simulink model "non_linear_model"  (R2023b)
settings: Solver=VariableStepAuto  StartTime=0.0  StopTime=6  RelTol=1e-3
values from neighbouring files (symbols this model uses):
  den_mag_C = Gden{1}    [Controllo_un_anello_v2.m]
  num_mag_C = Gnum{1}    [Controllo_un_anello_v2.m]
  Upper_bound_V = 23    [Controllo_un_anello_v2.m]
  x1_eq = 0.0044    [Controllo_un_anello_v2.m]
undefined symbols (not defined in the file or in its folder): k_mag, ki, kp, Lc, m, Rtot, theta, ueq, y0
libraries: slpidlib x2, SignalEditorBlockLib x1
settings Model: Creator=lollo  LastModifiedBy=lollo

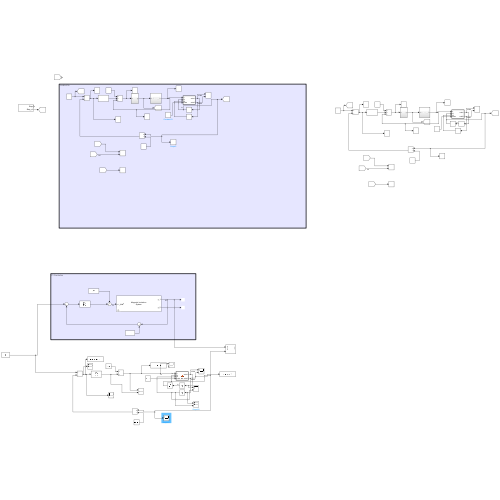
[thumbnail: Simulink's stored preview of the top-level diagram]
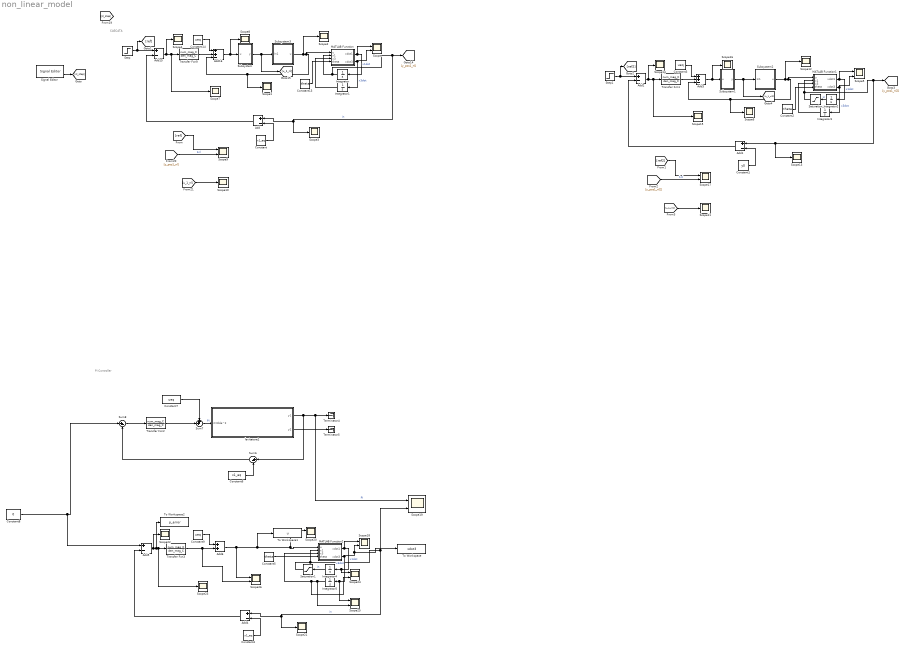
== system non_linear_model ==
  note: CASCATA
  note: PI Controller
  Add{,1..2,4..5,15} (6 alike) : Sum  Inputs=+-
  Add16 : Sum  Inputs=++-
  Add3 : Sum  Inputs=++-
  Add6 : Sum
  Constant : Constant  Value=x1_eq
  Constant1 : Constant  Value=y0
  Constant13 : Constant  Value=theta
  Constant{3,7,9,14} (4 alike) : Constant  Value=ueq
  Constant2 : Constant  Value=theta
  Constant4 : Constant  Value=x1_eq
  Constant5 : Constant  Value=theta
  Constant6 : Constant  Value=x1_eq
  Constant8 : Constant  Value=0
  Integrator{,1..5} (6 alike) : Integrator
  MATLAB Function : MATLAB Function  TreatAsAtomicUnit=on
  MATLAB Function1 : MATLAB Function  TreatAsAtomicUnit=on
  MATLAB Function2 : MATLAB Function  TreatAsAtomicUnit=on
  Saturation : Saturate  UpperLimit=0.012  LowerLimit=0
  Saturation1 : Saturate  UpperLimit=0.012  LowerLimit=0
  Scope{,5,9,17..20,24..26} (10 alike) : Scope  NumInputPorts=2
  Scope{1..4,6..8,10..16,21..23} (17 alike) : Scope
  Signal Editor : SignalEditorBlockLib/Signal Editor  FileName=input_signal.mat  ActiveScenario=Scenario  ActiveSignal=Step_nl  IsBus=off  OutputBusObjectStr=Bus: BusObject  SampleTime=0  Interpolate=off  ZeroCross=off  OutputAfterFinalValue=Setting to zero  Unit=inherit  PreserveSignalName=on  ApplySigPropsToAllScenarios=on  ApplySigPropsToAllSignals=off
  Step : Step  After=0.001  SampleTime=0
  Step1 : Step  After=0.001  SampleTime=0
  Subsystem : Subsystem
  Subsystem1 : Subsystem
  Subsystem2 : Subsystem
  Subsystem3 : Subsystem
  Sum6 : Sum  Inputs=|+-
  Sum7 : Sum  Inputs=++|
  Sum8 : Sum  Inputs=|+-
  Terminator4 : Terminator
  Terminator5 : Terminator
  To Workspace : ToWorkspace  VariableName=xdot3  SaveFormat=Timeseries  SampleTime=-1
  To Workspace1 : ToWorkspace  VariableName=u  SaveFormat=Timeseries  SampleTime=-1
  To Workspace2 : ToWorkspace  VariableName=p_error  SaveFormat=Timeseries  SampleTime=-1
  Transfer Fcn{1..3,9} (4 alike) : TransferFcn  Numerator=num_mag_C  Denominator=den_mag_C
  levitatore2 : Subsystem  Description=|  mask{y1_0=0, y2_0=0}
      | Magnetic Levitation System.
      | The input is the squared current. The outputs are the position (y1) and the velocity (y2).
      mask prompts: y1_0 "Initial value for y1"; y2_0 "Initial value for y2"
      mask DialogControl DescTextVar Prompt: Magnetic Levitation System. The input is the squared current. The outputs are the position (y1) and the velocity (y2).
      mask Display:
      | disp('Magnetic Levitation\nSystem');
      | port_label('input', 1, 'i= i\_tilde^2', 'texmode', 'on');
      | port_label('output', 1, 'y_1');
      | port_label('output', 2, 'y_2');
  wires:
  [y_pos1_nl] -> Scope9/2  "1nl"
  Transfer Fcn9/1 -> Add16/2
  Integrator/1 -> Add/1, Scope3/1, [y_pos1_nl], MATLAB Function/2(x1)  "in"
  Add16/1 -> Scope8/1, Subsystem/1(u)
  Integrator1/1 -> MATLAB Function/3(x3)
  Constant14/1 -> Add16/1
  Constant13/1 -> MATLAB Function/4(theta)
  Subsystem/1(y) -> [u_1_nl], Subsystem3/1(In1)
  MATLAB Function/1(xdot1) -> Scope/1, Integrator/1  "x1dot"
  Add15/1 -> Scope4/1, Scope7/1, Transfer Fcn9/1
  MATLAB Function/2(xdot3) -> Scope/2, Integrator1/1  "x3dot"
  [u_1_nl] -> Scope10/1
  Subsystem3/1(u) -> Scope2/1, MATLAB Function/1(u), Scope1/1, Add16/3
  Signal Editor/2 -> [nl_step]
  [ref] -> Scope9/1
  Step/1 -> [ref], Add15/1
  Constant/1 -> Add/2
  Add/1 -> Add15/2
  Add1/1 -> Add2/2
  Constant1/1 -> Add1/2
  [ref2] -> Scope17/1
  Subsystem2/1(u) -> Scope12/1, MATLAB Function1/1(u), Scope6/1, Add3/3
  [u_1_nl2] -> Scope11/1
  MATLAB Function1/1(xdot1) -> Scope5/1, Integrator2/1  "x1dot"
  Add2/1 -> Scope14/1, Scope15/1, Transfer Fcn1/1
  Constant3/1 -> Add3/1
  MATLAB Function1/2(xdot3) -> Scope5/2, Integrator3/1  "x3dot"
  Add3/1 -> Scope16/1, Subsystem1/1(u)
  Subsystem1/1(y) -> [u_1_nl2], Subsystem2/1(In1)
  Constant2/1 -> MATLAB Function1/4(theta)
  [y_pos1_nl2] -> Scope17/2  "1nl"
  Step1/1 -> [ref2], Add2/1
  Integrator3/1 -> MATLAB Function1/3(x3)
  Transfer Fcn1/1 -> Add3/2
  Integrator2/1 -> Saturation/1  "in"
  Saturation/1 -> Scope13/1, Add1/1, [y_pos1_nl2], MATLAB Function1/2(x1)
  levitatore2/1(y1) -> Sum6/1, Scope19/1, Terminator4/1  "PI"
  Sum6/1 -> Sum8/2
  levitatore2/2(y2) -> Terminator5/1
  Sum7/1 -> levitatore2/1(i=itilde^2)  "PI"
  Constant8/1 -> Add5/1, Sum8/1
  Sum8/1 -> Transfer Fcn2/1
  Constant6/1 -> Sum6/2
  Transfer Fcn2/1 -> Sum7/2
  Constant7/1 -> Sum7/1
  Add4/1 -> Add5/2
  Constant4/1 -> Add4/2
  Add6/1 -> Scope26/1, To Workspace1/1, MATLAB Function2/1(u), Scope20/1
  MATLAB Function2/1(xdot1) -> Scope18/1, Scope24/1, Integrator4/1  "x1dot"
  Add5/1 -> Scope22/1, To Workspace2/1, Scope23/1, Transfer Fcn3/1
  Constant9/1 -> Add6/1
  MATLAB Function2/2(xdot3) -> To Workspace/1, Scope18/2, Scope25/1, Integrator5/1  "x3dot"
  Constant5/1 -> MATLAB Function2/4(theta)
  Saturation1/1 -> Add4/1, Scope21/1, Scope19/2, MATLAB Function2/2(x1)  "in"
  Integrator5/1 -> Scope25/2, Scope24/2, MATLAB Function2/3(x3)
  Transfer Fcn3/1 -> Scope26/2, Add6/2
  Integrator4/1 -> Saturation1/1  "in"

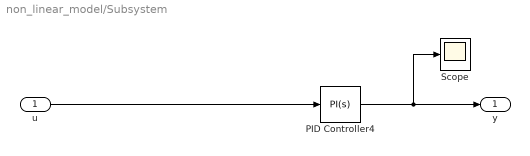
== system non_linear_model/Subsystem ==
  u : Inport
  PID Controller4 : slpidlib/PID Controller  Controller=PI  Form=Parallel  TimeDomain=Continuous-time  UseExternalTs=off  SampleTime=-1  IntegratorMethod=Forward Euler  FilterMethod=Forward Euler  ControllerParametersSource=internal  P=kp  I=ki  UseKiTs=off  D=0  N=100  UseFilter=on  TunerSelectOption=Transfer Function Based (PID Tuner App)  InitialConditionSource=internal  InitialConditionForIntegrator=0  InitialConditionForFilter=0  DifferentiatorICPrevScaledInput=0  ExternalReset=none  TrackingMode=off  Kt=1  LimitOutput=on  SatLimitsSource=internal  UpperSaturationLimit=Upper_bound_V  LowerSaturationLimit=0  LinearizeAsGain=on  AntiWindupMode=clamping  Kb=1  LimitIntegrator=off  UpperIntegratorSaturationLimit=inf  LowerIntegratorSaturationLimit=-inf  POutMin=[]  POutMax=[]  IOutMin=[]  IOutMax=[]  DOutMin=[]  DOutMax=[]  NOutMin=[]  NOutMax=[]  SumOutMin=[]  SumOutMax=[]  SaturationOutMin=[]  SaturationOutMax=[]  PParamMin=[]  PParamMax=[]  IParamMin=[]  IParamMax=[]  DParamMin=[]  DParamMax=[]  NParamMin=[]  NParamMax=[]  KbParamMin=[]  KbParamMax=[]  KtParamMin=[]  KtParamMax=[]  KbOutMin=[]  KbOutMax=[]  KtOutMin=[]  KtOutMax=[]  IntegratorOutMin=[]  IntegratorOutMax=[]  FilterOutMin=[]  FilterOutMax=[]  SumI1OutMin=[]  SumI1OutMax=[]  SumI2OutMin=[]  SumI2OutMax=[]  SumI3OutMin=[]  SumI3OutMax=[]  SumI4OutMin=[]  SumI4OutMax=[]  SumDOutMin=[]  SumDOutMax=[]  DifferentiatorOutMin=[]  DifferentiatorOutMax=[]  FilterDiffOutCoefMin=[]  FilterDiffOutCoefMax=[]  ReciprocalOutMin=[]  ReciprocalOutMax=[]  SumDenOutMin=[]  SumDenOutMax=[]  SumNumOutMin=[]  SumNumOutMax=[]  DivideOutMin=[]  DivideOutMax=[]  UdiffTsProdOutMin=[]  UdiffTsProdOutMax=[]  NTsProdOutMin=[]  NTsProdOutMax=[]  UintegralTsProdOutMin=[]  UintegralTsProdOutMax=[]  UngainTsProdOutMin=[]  UngainTsProdOutMax=[]  ClampingZeroOutDataTypeStr=Inherit: Inherit via back propagation  ClampingZeroOutMin=[]  ClampingZeroOutMax=[]  FilterDenConstantOutDataTypeStr=Inherit: Inherit via back propagation  FilterDenConstantOutMin=[]  FilterDenConstantOutMax=[]  PCopyOutDataTypeStr=Inherit: Inherit via back propagation  PCopyOutMin=[]  PCopyOutMax=[]  NCopyOutDataTypeStr=Inherit: Inherit via back propagation  NCopyOutMin=[]  NCopyOutMax=[]  IntegratorContinuousStateAttributes=''  IntegratorStateMustResolveToSignalObject=off  IntegratorRTWStateStorageClass=Auto  FilterContinuousStateAttributes=''  FilterStateMustResolveToSignalObject=off  FilterRTWStateStorageClass=Auto  ParallelPVariant=InternalParameters  IdealPVariant=Disabled  IVariant=InternalParameters  DVariant=Disabled  IntegratorVariant=Continuous  SatVariant=Enabled  AWVariant=ContClampingParallel  PCopyVariant=Disabled  TRVariant=Disabled  FdbkBlocksVariant=Forward  IdealPFdbkVariant=Disabled  SatFdbkVariant=Disabled  DerivativeFilterVariant=Disabled  NVariant=Disabled  NCopyVariant=Disabled_SignalSpec  FilterICVariant=Disabled  IntegratorICVariant=InternalICs  ExternalResetVariant=Disabled  TRSumVariant=Passthrough  SumFdbkVariant=Disabled  SumVariant=Sum_PI  TsampFilterVariant=InternalTs  TsampNgainVariant=Passthrough  TsampIntegralVariant=Disabled_SignalSpec  ExternalSaturationOutDataTypeStr=Inherit: Same as second input
  Scope : Scope
  y : Outport
  wires:
  PID Controller4/1 -> Scope/1, y/1
  u/1 -> PID Controller4/1

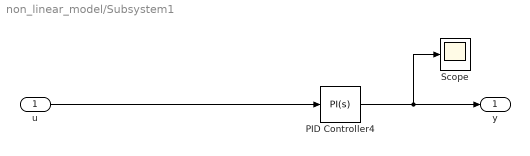
== system non_linear_model/Subsystem1 ==
  u : Inport
  PID Controller4 : slpidlib/PID Controller  Controller=PI  Form=Parallel  TimeDomain=Continuous-time  UseExternalTs=off  SampleTime=-1  IntegratorMethod=Forward Euler  FilterMethod=Forward Euler  ControllerParametersSource=internal  P=kp  I=ki  UseKiTs=off  D=0  N=100  UseFilter=on  TunerSelectOption=Transfer Function Based (PID Tuner App)  InitialConditionSource=internal  InitialConditionForIntegrator=0  InitialConditionForFilter=0  DifferentiatorICPrevScaledInput=0  ExternalReset=none  TrackingMode=off  Kt=1  LimitOutput=on  SatLimitsSource=internal  UpperSaturationLimit=Upper_bound_V  LowerSaturationLimit=0  LinearizeAsGain=on  AntiWindupMode=clamping  Kb=1  LimitIntegrator=off  UpperIntegratorSaturationLimit=inf  LowerIntegratorSaturationLimit=-inf  POutMin=[]  POutMax=[]  IOutMin=[]  IOutMax=[]  DOutMin=[]  DOutMax=[]  NOutMin=[]  NOutMax=[]  SumOutMin=[]  SumOutMax=[]  SaturationOutMin=[]  SaturationOutMax=[]  PParamMin=[]  PParamMax=[]  IParamMin=[]  IParamMax=[]  DParamMin=[]  DParamMax=[]  NParamMin=[]  NParamMax=[]  KbParamMin=[]  KbParamMax=[]  KtParamMin=[]  KtParamMax=[]  KbOutMin=[]  KbOutMax=[]  KtOutMin=[]  KtOutMax=[]  IntegratorOutMin=[]  IntegratorOutMax=[]  FilterOutMin=[]  FilterOutMax=[]  SumI1OutMin=[]  SumI1OutMax=[]  SumI2OutMin=[]  SumI2OutMax=[]  SumI3OutMin=[]  SumI3OutMax=[]  SumI4OutMin=[]  SumI4OutMax=[]  SumDOutMin=[]  SumDOutMax=[]  DifferentiatorOutMin=[]  DifferentiatorOutMax=[]  FilterDiffOutCoefMin=[]  FilterDiffOutCoefMax=[]  ReciprocalOutMin=[]  ReciprocalOutMax=[]  SumDenOutMin=[]  SumDenOutMax=[]  SumNumOutMin=[]  SumNumOutMax=[]  DivideOutMin=[]  DivideOutMax=[]  UdiffTsProdOutMin=[]  UdiffTsProdOutMax=[]  NTsProdOutMin=[]  NTsProdOutMax=[]  UintegralTsProdOutMin=[]  UintegralTsProdOutMax=[]  UngainTsProdOutMin=[]  UngainTsProdOutMax=[]  ClampingZeroOutDataTypeStr=Inherit: Inherit via back propagation  ClampingZeroOutMin=[]  ClampingZeroOutMax=[]  FilterDenConstantOutDataTypeStr=Inherit: Inherit via back propagation  FilterDenConstantOutMin=[]  FilterDenConstantOutMax=[]  PCopyOutDataTypeStr=Inherit: Inherit via back propagation  PCopyOutMin=[]  PCopyOutMax=[]  NCopyOutDataTypeStr=Inherit: Inherit via back propagation  NCopyOutMin=[]  NCopyOutMax=[]  IntegratorContinuousStateAttributes=''  IntegratorStateMustResolveToSignalObject=off  IntegratorRTWStateStorageClass=Auto  FilterContinuousStateAttributes=''  FilterStateMustResolveToSignalObject=off  FilterRTWStateStorageClass=Auto  ParallelPVariant=InternalParameters  IdealPVariant=Disabled  IVariant=InternalParameters  DVariant=Disabled  IntegratorVariant=Continuous  SatVariant=Enabled  AWVariant=ContClampingParallel  PCopyVariant=Disabled  TRVariant=Disabled  FdbkBlocksVariant=Forward  IdealPFdbkVariant=Disabled  SatFdbkVariant=Disabled  DerivativeFilterVariant=Disabled  NVariant=Disabled  NCopyVariant=Disabled_SignalSpec  FilterICVariant=Disabled  IntegratorICVariant=InternalICs  ExternalResetVariant=Disabled  TRSumVariant=Passthrough  SumFdbkVariant=Disabled  SumVariant=Sum_PI  TsampFilterVariant=InternalTs  TsampNgainVariant=Passthrough  TsampIntegralVariant=Disabled_SignalSpec  ExternalSaturationOutDataTypeStr=Inherit: Same as second input
  Scope : Scope
  y : Outport
  wires:
  PID Controller4/1 -> Scope/1, y/1
  u/1 -> PID Controller4/1

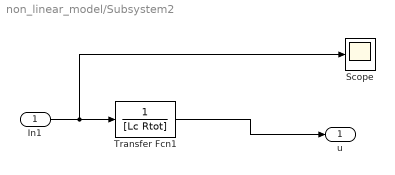
== system non_linear_model/Subsystem2 ==
  In1 : Inport
  Scope : Scope
  Transfer Fcn1 : TransferFcn  Denominator=[Lc Rtot]
  u : Outport
  wires:
  In1/1 -> Scope/1, Transfer Fcn1/1
  Transfer Fcn1/1 -> u/1

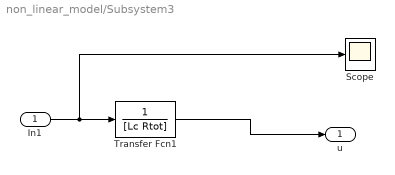
== system non_linear_model/Subsystem3 ==
  In1 : Inport
  Scope : Scope
  Transfer Fcn1 : TransferFcn  Denominator=[Lc Rtot]
  u : Outport
  wires:
  In1/1 -> Scope/1, Transfer Fcn1/1
  Transfer Fcn1/1 -> u/1

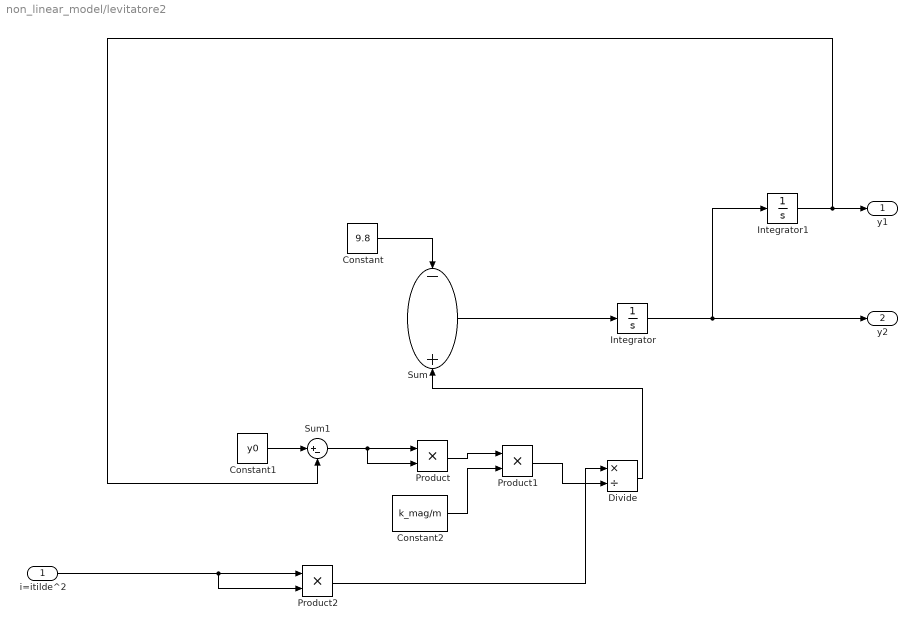
== system non_linear_model/levitatore2 ==
  i=itilde^2 : Inport
  Constant : Constant  Value=9.8
  Constant1 : Constant  Value=y0
  Constant2 : Constant  Value=k_mag/m
  Divide : Product  Inputs=*/
  Integrator : Integrator  InitialCondition=y2_0
  Integrator1 : Integrator  InitialCondition=y1_0
  Product : Product  RndMeth=Zero
  Product1 : Product  RndMeth=Zero
  Product2 : Product  RndMeth=Zero
  Sum : Sum  Inputs=-+
  Sum1 : Sum  Inputs=|+-
  y1 : Outport
  y2 : Outport  Port=2
  wires:
  Constant/1 -> Sum/1
  Constant1/1 -> Sum1/1
  Sum1/1 -> Product/1, Product/2
  Product/1 -> Product1/1
  Constant2/1 -> Product1/2
  Product1/1 -> Divide/2
  Divide/1 -> Sum/2
  Sum/1 -> Integrator/1
  Integrator/1 -> Integrator1/1, y2/1
  Integrator1/1 -> Sum1/2, y1/1
  Product2/1 -> Divide/1
  i=itilde^2/1 -> Product2/2, Product2/1

== matlab function non_linear_model/MATLAB Function1 ==
  data: u input; xdot1 output; x1 input; x3 input; xdot3 output; theta input
function [xdot1, xdot3] = fcn(u, x1, x3, theta)
    k_aero = theta(1, 1);
    k_mag = theta(2, 1);
    m = theta(3, 1);
    y0 = theta(4, 1);
    Rtot = theta(5, 1);
    Lc = theta(6, 1);
    g = 9.81;


    xdot1 = x3;


    xdot3 = (k_mag/m) * (u / (y0 - x1+eps))^2 - g;

== matlab function non_linear_model/MATLAB Function ==
  data: u input; xdot1 output; x1 input; x3 input; xdot3 output; theta input
function [xdot1, xdot3] = fcn(u, x1, x3, theta)
    k_aero = theta(1, 1);
    k_mag = theta(2, 1);
    m = theta(3, 1);
    y0 = theta(4, 1);
    Rtot = theta(5, 1);
    Lc = theta(6, 1);
    g = 9.81;

    if x1<=0 && x3<0
        x1 = 0;
        xdot1 = 0;
        
    elseif x1>=y0 && x3>0
        x1 = y0-eps;
        xdot1 = 0;
    else
        xdot1 = x3;

    end
    

xdot3 = (k_mag/m) * (u / (y0 - x1))^2 - g;

== matlab function non_linear_model/MATLAB Function2 ==
  data: u input; xdot1 output; x1 input; x3 input; xdot3 output; theta input
function [xdot1, xdot3] = fcn(u, x1, x3, theta)
    k_aero = theta(1, 1);
    k_mag = theta(2, 1);
    m = theta(3, 1);
    y0 = theta(4, 1);
    Rtot = theta(5, 1);
    Lc = theta(6, 1);
    g = 9.81;
    xdot3 = (k_mag/m) * (u / (y0 - x1))^2 - g;
    if x1<=0 && x3<=0 && xdot3<0
        x1 = 0;
        xdot1 = 0;
        xdot3 = 0;
        
    elseif x1>=y0 && x3>0
        x1 = y0-eps;
        xdot1 = 0;
        xdot3 = 0;
    else
        xdot1 = x3;
        

    end
